simulink model "exampleWetherFromFile"  (Simulink 7.6)
settings: Solver=ode45  StartTime=90*24*3600  StopTime=100*24*3600  RelTol=1e-3
libraries: carnot x1
settings Model: Creator=drhf  LastModifiedBy=drhf
settings CodeAppCC: CustomSymbolStrType=$N$R$M_T

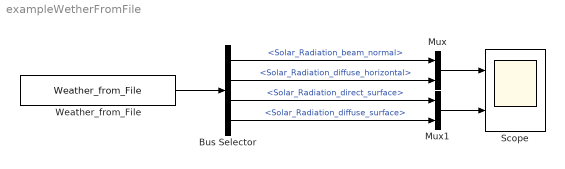
== system exampleWetherFromFile ==
  Bus Selector : BusSelector  OutputSignals=Solar_Radiation_beam_normal,Solar_Radiation_diffuse_horizontal,Solar_Radiation_direct_surface,Solar_Radiation_diffuse_surface
  Mux : Mux  Inputs=2
  Mux1 : Mux  Inputs=2
  Scope : Scope  NumInputPorts=2
      settings: YMin=-5~-5  YMax=5~5
  Weather_from_File : carnot/Weather/Weather_from_File  SystemSampleTime=-1  file=DE_TRY2010_06_averageYear  ext=.mat
  wires:
  Weather_from_File/1 -> Bus Selector/1
  Bus Selector/1 -> Mux/1  "<Solar_Radiation_beam_normal>"
  Bus Selector/2 -> Mux/2  "<Solar_Radiation_diffuse_horizontal>"
  Bus Selector/3 -> Mux1/1  "<Solar_Radiation_direct_surface>"
  Bus Selector/4 -> Mux1/2  "<Solar_Radiation_diffuse_surface>"
  Mux/1 -> Scope/1
  Mux1/1 -> Scope/2
